simulink model "third"  (R2012b)
settings: Solver=ode45  SolverMode=SingleTasking  StartTime=0.0  StopTime=10.0  RelTol=1e-3
libraries: simulink x1
settings Model: CovMetricSettings=dwe  CovHtmlReporting=off  covSaveCumulativeToWorkspaceVar=off  CovSaveSingleToWorkspaceVar=off  CovExternalEMLEnable=on  Creator=Pranshu  LastModifiedBy=Pranshu
settings DataIOCC: LimitDataPoints=off  SaveFormat=StructureWithTime  ReturnWorkspaceOutputs=on
settings OptimizationCC: ExpressionDepthLimit=128
settings DebuggingCC: UnderspecifiedInitializationDetection=Simplified  MergeDetectMultiDrivingBlocksExec=error  SolverPrmCheckMsg=none  FrameProcessingCompatibilityMsg=error  StateNameClashWarn=none  SFUnexpectedBacktrackingDiag=error  SFNoUnconditionalDefaultTransitionDiag=error
settings HardwareCC: ProdBitPerPointer=64  ProdLargestAtomicFloat=Float  ProdIntDivRoundTo=Zero  ProdEndianess=LittleEndian  ProdHWDeviceType=Specified
settings ModelReferenceCC: PropagateSignalLabelsOutOfModel=on
settings SFSimCC: SimUseLocalCustomCode=on
settings RTWCC: RTWUseLocalCustomCode=on
settings CodeAppCC: CustomSymbolStrType=$N$R$M_T
settings GRTTargetCC: CodeReplacementLibrary=C99 (ISO)  GeneratePreprocessorConditionals=Use local settings

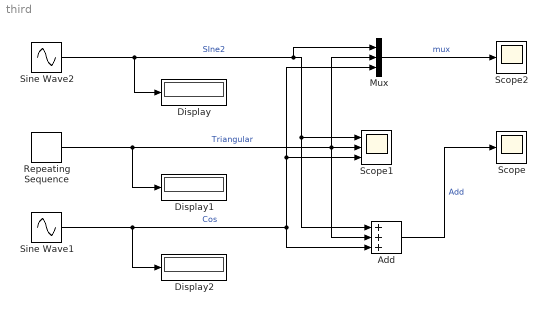
== system third ==
  Add : Sum  Inputs=+++
  Display : Display
  Display1 : Display
  Display2 : Display
  Mux : Mux  Inputs=3
  Repeating Sequence : simulink/Sources/Repeating Sequence  rep_seq_t=[0 2]  rep_seq_y=[0 5]
  Scope : Scope
      settings: TimeRange=auto  ShowLegends=on  MaxDataPoints=5000  SaveToWorkspace=off  SaveName=ScopeData  YMin=-5.02617  YMax=9.45712  SampleTime=-1
  Scope1 : Scope  NumInputPorts=3
      settings: TimeRange=auto  ShowLegends=on  MaxDataPoints=5000  SaveToWorkspace=off  YMin=-3.92704~-3.92704~-3.92704  YMax=5.43634~5.43634~5.43634  SampleTime=-1
  Scope2 : Scope
      settings: TimeRange=auto  ShowLegends=on  MaxDataPoints=5000  SaveToWorkspace=off  SaveName=ScopeData2  YMin=-3.92704  YMax=5.43634  SampleTime=-1
  Sine Wave1 : Sin  Amplitude=2  Frequency=2  Phase=1.5707  SampleTime=0
  Sine Wave2 : Sin  Amplitude=3  Frequency=2  SampleTime=0
  wires:
  Repeating Sequence/1 -> Display1/1, Mux/2, Add/2, Scope1/2  "Triangular"
  Sine Wave2/1 -> Display/1, Mux/1, Add/1, Scope1/1  "SIne2"
  Sine Wave1/1 -> Display2/1, Mux/3, Scope1/3, Add/3  "Cos"
  Add/1 -> Scope/1  "Add"
  Mux/1 -> Scope2/1  "mux"
